simulink model "BasicEnergyBalancePlant"  (R2024b)
settings: Solver=VariableStepAuto  StartTime=0.0  StopTime=10.0  RelTol=1e-3
undefined symbols (not defined in the file): Cm, Rth
settings Model: Creator=joshr  LastModifiedBy=joshr

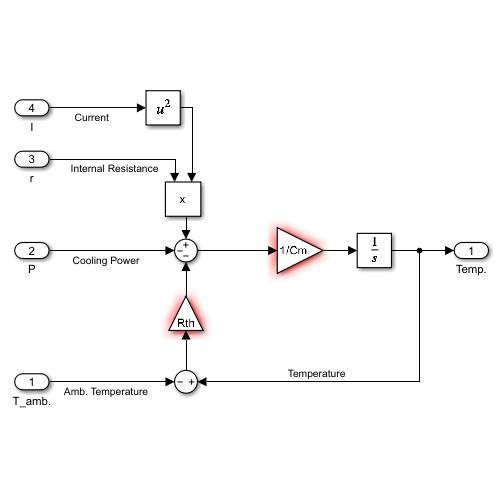
[thumbnail: Simulink's stored preview of the top-level diagram]
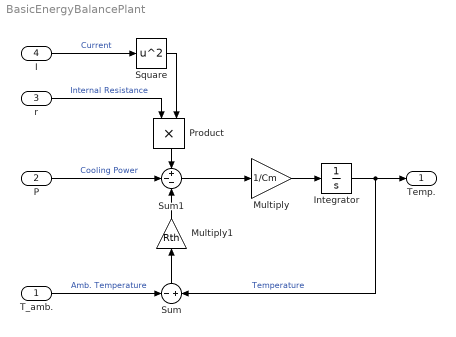
== system BasicEnergyBalancePlant ==
  T_amb. : Inport
  P : Inport  Port=2
  r : Inport  Port=3
  I : Inport  Port=4
  Integrator : Integrator
  Multiply : Gain  Gain=1/Cm
  Multiply1 : Gain  Gain=Rth
  Product : Product
  Square : Math  Operator=square
  Sum : Sum  Inputs=-+
  Sum1 : Sum  Inputs=+--
  Temp. : Outport
  wires:
  Multiply/1 -> Integrator/1
  Integrator/1 -> Temp./1, Sum/2  "Temperature"
  Sum/1 -> Multiply1/1
  T_amb./1 -> Sum/1  "Amb. Temperature"
  Multiply1/1 -> Sum1/3
  Sum1/1 -> Multiply/1
  P/1 -> Sum1/2  "Cooling Power"
  r/1 -> Product/1  "Internal Resistance"
  I/1 -> Square/1  "Current"
  Square/1 -> Product/2
  Product/1 -> Sum1/1
